simulink model "Flux_Nonsensor"  (R2024a)
settings: Solver=FixedStepDiscrete  StartTime=0.0  StopTime=2  FixedStep=Fixed_Step_Size  RelTol=1e-3
InitFcn:
  | Flux_Nonsensor_data_new
  | 
  | supplyVoltage=30;
values from neighbouring files (symbols this model uses):
  A = 1    [saddleToDuty.m]
  BandwidthCurrentPI = 1256*1.5    (= 1884)    [Flux_Nonsensor_data_new.m]
  Fixed_Step_Size = 1e-6    (= 1e-06)    [Flux_Nonsensor_data_new.m]
  Flux = 0.01837    [Flux_Nonsensor_data_new.m]
  Gamma = mpt.Parameter    [Flux_Nonsensor_data_new.m]
  Ld = 0.0001    [Flux_Nonsensor_data_new.m]
  Lq = 0.0001040    (= 0.000104)    [Flux_Nonsensor_data_new.m]
  Ls = 0.000195185    [Flux_Nonsensor_data_new.m]
  MaxVoltage = 10    [Flux_Nonsensor_data_new.m]
  pll_omega = mpt.Parameter    [Flux_Nonsensor_data_new.m]
  pll_xi = mpt.Parameter    [Flux_Nonsensor_data_new.m]
  PolePairs = 3    [Flux_Nonsensor_data_new.m]
  Rs = 0.02065    [Flux_Nonsensor_data_new.m]
  Speed_Ki = mpt.Parameter    [Flux_Nonsensor_data_new.m]
  Speed_Kp = mpt.Parameter    [Flux_Nonsensor_data_new.m]
  Speed_PI_OutputMax = 8    [Flux_Nonsensor_data_new.m]
  Speed_PI_OutputMin = -8    [Flux_Nonsensor_data_new.m]
  TsBSP = 1e-4    (= 0.0001)    [Flux_Nonsensor_data_new.m]
  TsBSP_MODEL = 2.5e-5    (= 2.5e-05)    [Flux_Nonsensor_data_new.m]
  TsFOC = 1e-4    (= 0.0001)    [Flux_Nonsensor_data_new.m]
undefined symbols (not defined in the file or in its folder): DiscIntNeverNeededParam, magnitude
libraries: slpidlib x3, simulink x2, mcbplantlib x1, spsDCVoltageSourceLib x1, spsSVPWMGenerator2LevelLib x1, spsGroundLib x1, autolibpmsminterior x1, spsPermanentMagnetSynchronousMachineLib x1, spsThreePhaseVIMeasurementLib x1, spsUniversalBridgeLib x1, spspowerguiLib x1
(part 2 of 2)

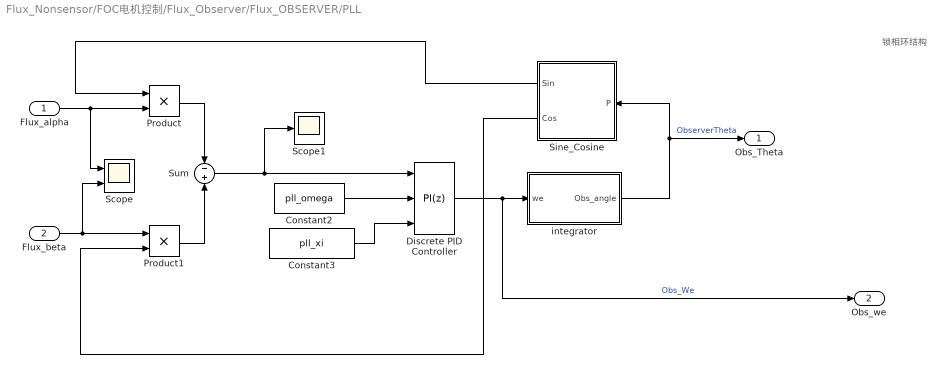
== system Flux_Nonsensor/FOC电机控制/Flux_Observer/Flux_OBSERVER/PLL ==
  note: 锁相环结构
  Flux_alpha : Inport  OutDataTypeStr=single
  Flux_beta : Inport  Port=2  OutDataTypeStr=single
  Constant2 : Constant  Value=pll_omega  OutDataTypeStr=single
  Constant3 : Constant  Value=pll_xi  OutDataTypeStr=single
  Discrete PID Controller : slpidlib/PID Controller  Controller=PI  Form=Parallel  TimeDomain=Discrete-time  UseExternalTs=off  SampleTime=-1  IntegratorMethod=Forward Euler  FilterMethod=Forward Euler  ControllerParametersSource=external  P=2*0.707*1650  I=1650*1650  UseKiTs=off  D=0  UseExternalDerivativeSource=off  N=100  UseFilter=on  TunerSelectOption=Transfer Function Based (PID Tuner App)  ZeroCross=off  InitialConditionSource=internal  InitialConditionForIntegrator=0  InitialConditionForFilter=0  DifferentiatorICPrevScaledInput=0  ExternalReset=none  TrackingMode=off  Kt=1  LimitOutput=on  SatLimitsSource=internal  UpperSaturationLimit=3000*2*pi*PolePairs/60  LowerSaturationLimit=-3000*2*pi*PolePairs/60  LinearizeAsGain=off  AntiWindupMode=clamping  Kb=1  LimitIntegrator=off  UpperIntegratorSaturationLimit=inf  LowerIntegratorSaturationLimit=-inf  POutMin=[]  POutMax=[]  IOutMin=[]  IOutMax=[]  DOutMin=[]  DOutMax=[]  NOutMin=[]  NOutMax=[]  SumOutMin=[]  SumOutMax=[]  SaturationOutMin=[]  SaturationOutMax=[]  PParamMin=[]  PParamMax=[]  IParamMin=[]  IParamMax=[]  DParamMin=[]  DParamMax=[]  NParamMin=[]  NParamMax=[]  KbParamMin=[]  KbParamMax=[]  KtParamMin=[]  KtParamMax=[]  KbOutMin=[]  KbOutMax=[]  KtOutMin=[]  KtOutMax=[]  IntegratorOutMin=[]  IntegratorOutMax=[]  FilterOutMin=[]  FilterOutMax=[]  SumI1OutMin=[]  SumI1OutMax=[]  SumI2OutMin=[]  SumI2OutMax=[]  SumI3OutMin=[]  SumI3OutMax=[]  SumI4OutMin=[]  SumI4OutMax=[]  SumDOutMin=[]  SumDOutMax=[]  DifferentiatorOutMin=[]  DifferentiatorOutMax=[]  FilterDiffOutCoefMin=[]  FilterDiffOutCoefMax=[]  ReciprocalOutMin=[]  ReciprocalOutMax=[]  SumDenOutMin=[]  SumDenOutMax=[]  SumNumOutMin=[]  SumNumOutMax=[]  DivideOutMin=[]  DivideOutMax=[]  UdiffTsProdOutMin=[]  UdiffTsProdOutMax=[]  NTsProdOutMin=[]  NTsProdOutMax=[]  UintegralTsProdOutMin=[]  UintegralTsProdOutMax=[]  UngainTsProdOutMin=[]  UngainTsProdOutMax=[]  ClampingZeroOutDataTypeStr=Inherit: Inherit via back propagation  ClampingZeroOutMin=[]  ClampingZeroOutMax=[]  FilterDenConstantOutDataTypeStr=Inherit: Inherit via back propagation  FilterDenConstantOutMin=[]  FilterDenConstantOutMax=[]  PCopyOutDataTypeStr=Inherit: Inherit via back propagation  PCopyOutMin=[]  PCopyOutMax=[]  NCopyOutDataTypeStr=Inherit: Inherit via back propagation  NCopyOutMin=[]  NCopyOutMax=[]  IntegratorContinuousStateAttributes=''  IntegratorStateMustResolveToSignalObject=off  IntegratorRTWStateStorageClass=Auto  FilterContinuousStateAttributes=''  FilterStateMustResolveToSignalObject=off  FilterRTWStateStorageClass=Auto  ParallelPVariant=ExternalParameters  IdealPVariant=Disabled  IVariant=ExternalParameters  DVariant=Disabled  IntegratorVariant=Discrete  SatVariant=Enabled  AWVariant=DiscClampingParallel  PCopyVariant=Disabled  TRVariant=Disabled  FdbkBlocksVariant=Forward  IdealPFdbkVariant=Disabled  SatFdbkVariant=Disabled  DerivativeFilterVariant=Disabled  NVariant=Disabled  NCopyVariant=Disabled_SignalSpec  FilterICVariant=Disabled  IntegratorICVariant=InternalICs  ExternalResetVariant=Disabled  TRSumVariant=Passthrough  SumFdbkVariant=Disabled  SumVariant=Sum_PI  TsampFilterVariant=InternalTs  TsampNgainVariant=Passthrough  TsampIntegralVariant=Disabled_SignalSpec  ExternalSaturationOutDataTypeStr=Inherit: Same as second input  DerivativeSourceVariant=Disabled
  Product : Product  OutDataTypeStr=single
  Product1 : Product  OutDataTypeStr=single
  Scope : Scope  NumInputPorts=2
  Scope1 : Scope
  Sine_Cosine : Subsystem  TreatAsAtomicUnit=on
      settings: RTWSystemCode=Nonreusable function  RTWFcnNameOpts=Use subsystem name
  Sum : Sum  Inputs=-|+  OutDataTypeStr=single
  integrator : Subsystem
  Obs_Theta : Outport  OutDataTypeStr=single
  Obs_we : Outport  Port=2  OutDataTypeStr=single
  wires:
  Product/1 -> Sum/1
  Product1/1 -> Sum/2
  Sum/1 -> Scope1/1, Discrete PID Controller/1
  Sine_Cosine/2(Cos) -> Product1/2
  Sine_Cosine/1(Sin) -> Product/1
  integrator/1(Obs_angle) -> Obs_Theta/1, Sine_Cosine/1(P)  "ObserverTheta"
  Flux_alpha/1 -> Scope/1, Product/2
  Flux_beta/1 -> Scope/2, Product1/1
  Discrete PID Controller/1 -> Obs_we/1, integrator/1(we)  "Obs_We"
  Constant3/1 -> Discrete PID Controller/3
  Constant2/1 -> Discrete PID Controller/2

== system Flux_Nonsensor/FOC电机控制/Flux_Observer/Flux_OBSERVER/PLL/Sine_Cosine ==
  note: Sine Cosine Coefficients
  P : Inport  OutDataTypeStr=single
  Cos1 : Trigonometry  Operator=cos
  Saturation : Saturate  UpperLimit=2*pi-0.001  LowerLimit=0+0.001  OutDataTypeStr=single
  Scope : Scope  NumInputPorts=2
  Sin1 : Trigonometry
  Sin : Outport  VectorParamsAs1DForOutWhenUnconnected=off
  Cos : Outport  Port=2  VectorParamsAs1DForOutWhenUnconnected=off
  wires:
  P/1 -> Saturation/1  "position"
  Sin1/1 -> Scope/1, Sin/1
  Cos1/1 -> Scope/2, Cos/1
  Saturation/1 -> Cos1/1, Sin1/1

== system Flux_Nonsensor/FOC电机控制/Flux_Observer/Flux_OBSERVER/PLL/integrator ==
  we : Inport  OutDataTypeStr=single
  Angle_Limit : Subsystem
  Sum1 : Sum  Inputs=|++  OutDataTypeStr=single
  Ts : Gain  Gain=TsFOC  OutDataTypeStr=single
  Unit Delay : UnitDelay  SampleTime=-1  HasFrameUpgradeWarning=on
  Obs_angle : Outport  OutDataTypeStr=single
  wires:
  we/1 -> Ts/1
  Ts/1 -> Sum1/1
  Sum1/1 -> Angle_Limit/1(Angle_input)
  Unit Delay/1 -> Obs_angle/1, Sum1/2
  Angle_Limit/1(Angle_output) -> Unit Delay/1

== system Flux_Nonsensor/FOC电机控制/Flux_Observer/Flux_OBSERVER/PLL/integrator/Angle_Limit ==
  Angle_input : Inport
  If Action Subsystem1 : Subsystem  TreatAsAtomicUnit=on
  If Action Subsystem2 : Subsystem  TreatAsAtomicUnit=on
  If Action Subsystem3 : Subsystem  TreatAsAtomicUnit=on
  If1 : If  IfExpression=u1 > 6.283185307  ElseIfExpressions=u1<0
  Merge1 : Merge  Inputs=3
  Angle_output : Outport
  wires:
  If1/2 -> If Action Subsystem3/Action
  If1/1 -> If Action Subsystem2/Action
  If1/3 -> If Action Subsystem1/Action
  Merge1/1 -> Angle_output/1
  If Action Subsystem1/1(Out1) -> Merge1/3
  If Action Subsystem2/1(Out1) -> Merge1/1
  Angle_input/1 -> If Action Subsystem3/1(In1), If Action Subsystem1/1(In1), If Action Subsystem2/1(In1), If1/1
  If Action Subsystem3/1(Out1) -> Merge1/2

== system Flux_Nonsensor/FOC电机控制/Flux_Observer/Flux_OBSERVER/PLL/integrator/Angle_Limit/If Action Subsystem1 ==
  In1 : Inport
  Action Port : ActionPort  ActionPortLabel=else
  Out1 : Outport
  wires:
  In1/1 -> Out1/1

== system Flux_Nonsensor/FOC电机控制/Flux_Observer/Flux_OBSERVER/PLL/integrator/Angle_Limit/If Action Subsystem2 ==
  In1 : Inport
  Action Port : ActionPort  ActionPortLabel=if(u1 > 6.283185307)
  2pi : Constant  Value=2*pi  OutDataTypeStr=single
  Subtract1 : Sum  Inputs=+-  OutDataTypeStr=single
  Out1 : Outport
  wires:
  In1/1 -> Subtract1/1
  Subtract1/1 -> Out1/1
  2pi/1 -> Subtract1/2

== system Flux_Nonsensor/FOC电机控制/Flux_Observer/Flux_OBSERVER/PLL/integrator/Angle_Limit/If Action Subsystem3 ==
  In1 : Inport
  Action Port : ActionPort  ActionPortLabel=elseif(u1<0)
  Angle_offset : Constant  Value=2*pi  OutDataTypeStr=single
  Subtract1 : Sum
  Out1 : Outport
  wires:
  In1/1 -> Subtract1/1
  Subtract1/1 -> Out1/1
  Angle_offset/1 -> Subtract1/2

== matlab function Flux_Nonsensor/FOC电机控制/MATLAB Function ==
  data: saddle1 input; saddle2 input; saddle3 input; frequency input; pwm1 output; deadtime input; pwm1_comp output; pwm2 output; pwm2_comp output; pwm3 output; pwm3_comp output
function [pwm1, pwm1_comp, pwm2, pwm2_comp, pwm3, pwm3_comp] = generatePWMDuty(saddle1, saddle2, saddle3, frequency, deadtime)
    % 参数说明：
    % saddle1, saddle2, saddle3: 输入的三个马鞍波信号（归一化0-1）
    % frequency: PWM 的频率，单位 Hz
    % deadtime: 死区时间，单位 us
    
    % 检查输入信号长度一致性
    if length(saddle1) ~= length(saddle2) || length(saddle2) ~= length(saddle3)
        %error('输入的三个马鞍波信号长度必须一致');
    end
    
    % 设定仿真参数
    Ts = 1e-6; % 仿真步长，1微秒
    T_pwm = 1 / frequency; % PWM周期
    t = (0:length(saddle1)-1) * Ts; % 时间轴与信号点一致
    
    % 生成三角波（0-1归一化）
    triangle = mod(t / T_pwm, 1);
    
    % 比较生成PWM信号
    pwm1 = saddle1 > triangle;
    pwm2 = saddle2 > triangle;
    pwm3 = saddle3 > triangle;
    
    % 生成互补PWM信号
    pwm1_comp = ~pwm1;
    pwm2_comp = ~pwm2;
    pwm3_comp = ~pwm3;
    
    % 添加死区
    deadtime_steps = round(deadtime / (Ts * 1e6)); % 死区转换为步数
    pwm1 = addDeadtime(pwm1, pwm1_comp, deadtime_steps);
    pwm2 = addDeadtime(pwm2, pwm2_comp, deadtime_steps);
    pwm3 = addDeadtime(pwm3, pwm3_comp, deadtime_steps);
    
    % 输出
    pwm1_comp = ~pwm1; % 更新互补波
    pwm2_comp = ~pwm2;
    pwm3_comp = ~pwm3;
end

function pwm_out = addDeadtime(pwm, pwm_comp, deadtime_steps)
    % 为PWM信号添加死区时间
    pwm_out = pwm;
    for i = 1:length(pwm) - deadtime_steps
        if pwm(i) && pwm_comp(i + deadtime_steps)
            pwm_out(i:i + deadtime_steps) = 0;
        end
    end
end

== matlab function Flux_Nonsensor/FOC电机控制/SVPWM MATLAB Function ==
  data: Valpha input single size=1; Tcmp1 output single size=1; Vbeta input single size=1; Tcmp2 output single size=1; Tcmp3 output single size=1; Udc input single size=1; Tpwm input single size=1; sector output single size=1
function [Tcmp1,Tcmp2,Tcmp3,sector] = fcn(Valpha,Vbeta,Udc,Tpwm)
%#codegen

sector = single(0);
Tcmp1 = single(0);
Tcmp2 = single(0);
Tcmp3 = single(0);

%========Parameters statement================

    Vref1 = Vbeta;							                   
    Vref2 = (sqrt(3)*Valpha - Vbeta)/2; 				    
    Vref3 = (-sqrt(3)*Valpha - Vbeta)/2;					
   
 %========Sector calculation=================

  if (Vref1>0)
	   sector = single(1);
  end
  if (Vref2>0)
	   sector = sector+single(2);
  end
  if (Vref3>0)
       sector = sector+single(4);
  end

%======== X Y Z calculation===================

X = sqrt(3)*Vbeta*Tpwm/Udc;
Y = Tpwm/Udc*(3/2*Valpha+sqrt(3)/2*Vbeta);
Z = Tpwm/Udc*(-3/2*Valpha+sqrt(3)/2*Vbeta);	         

%==========Duty ratio calculation================
switch (sector)   
    case 1
        T1 = Z; T2 = Y; 
	case 2
        T1 = Y; T2 = -X; 
	case 3
        T1 = -Z; T2 = X; 
	case 4
        T1 = -X; T2 = Z;
	case 5
        T1 = X; T2 = -Y;
    otherwise
        T1 = -Y; T2 = -Z;
end

if T1+T2 > Tpwm
    T1 = T1/(T1+T2);
    T2 = T2/(T1+T2);
else
    T1 = T1;
    T2 = T2;
end
ta = (Tpwm-(T1+T2))/4.0;
tb = ta+T1/2;
tc = tb+T2/2;

%==========Duty ratio calculation================
switch (sector)
    case 1 
        Tcmp1=tb;
        Tcmp2=ta;
        Tcmp3=tc; 
        
    case 2 
        Tcmp1=ta;
        Tcmp2=tc;
        Tcmp3=tb; 
       
    case 3 
        Tcmp1=ta;
        Tcmp2=tb;
        Tcmp3=tc; 
        
    case 4 
        Tcmp1=tc;
        Tcmp2=tb;
        Tcmp3=ta;
        
    case 5 
        Tcmp1=tc;
        Tcmp2=ta;
        Tcmp3=tb;
        
   case 6
       Tcmp1=tb;
       Tcmp2=tc;
       Tcmp3=ta;
end
end

== matlab function Flux_Nonsensor/FOC电机控制/MATLAB Function1 ==
  data: Valpha input; duty_3 output; Vbeta input; Vdc input
function duty_3 = svGen(Valpha,Vbeta,Vdc)
Valpha_Pu = Valpha/Vdc;
Vbeta_Pu = Vbeta/Vdc;
Vabc_Pu = zeros(3,1);
duty = zeros(3,1);

Vabc_Pu(1) = Valpha_Pu;
Vabc_Pu(2) = -0.5*Valpha_Pu + sqrt(3)/2 * Vbeta_Pu;
Vabc_Pu(3) = -0.5*Valpha_Pu - sqrt(3)/2 * Vbeta_Pu;

Vmax_Pu = max(Vabc_Pu);
Vmin_Pu = min(Vabc_Pu);

Vcom_Pu =0.5 *(Vmax_Pu + Vmin_Pu);

duty(1) = Vabc_Pu(1) - Vcom_Pu + 0.5;
duty(2) = Vabc_Pu(2) - Vcom_Pu + 0.5;
duty(3) = Vabc_Pu(3) - Vcom_Pu + 0.5;
duty_3 = duty;

== matlab function Flux_Nonsensor/MATLAB Function ==
  data: waveA input; pwmHighA output; waveB input; waveC input; samplingInterval input; switchFreq input; deadTime input; pwmLowA output; pwmHighB output; pwmLowB output; pwmHighC output; pwmLowC output
function [pwmHighA, pwmLowA, pwmHighB, pwmLowB, pwmHighC, pwmLowC] = generatePWM6(waveA, waveB, waveC, samplingInterval, switchFreq, deadTime)
    % 参数说明：
    % waveA, waveB, waveC: 输入的三个马鞍波信号 (离散数组)
    % samplingInterval: 最小采样间隔（秒），如 100e-6
    % switchFreq: MOSFET 切换频率 (Hz)
    % deadTime: 死区时间（秒），如 1e-6

    % 计算 PWM 的基准周期
    pwmPeriod = 1 / switchFreq;        % PWM周期 (秒)
    samplesPerCycle = round(pwmPeriod / samplingInterval); % 每个周期的采样点数
    deadSamples = round(deadTime / samplingInterval);      % 死区对应的采样点数

    % 将输入波形归一化到 [0, 1] 区间
    waveA = normalizeWave(waveA);
    waveB = normalizeWave(waveB);
    waveC = normalizeWave(waveC);

    % 生成每对PWM波形
    [pwmHighA, pwmLowA] = createPWM(waveA, samplesPerCycle, deadSamples);
    [pwmHighB, pwmLowB] = createPWM(waveB, samplesPerCycle, deadSamples);
    [pwmHighC, pwmLowC] = createPWM(waveC, samplesPerCycle, deadSamples);
end

function normalizedWave = normalizeWave(wave)
    % 将波形归一化到 [0, 1] 区间
    minVal = min(wave);
    maxVal = max(wave);
    normalizedWave = (wave - minVal) / (maxVal - minVal);
end

function [pwmHigh, pwmLow] = createPWM(wave, samplesPerCycle, deadSamples)
    % 根据输入波形生成一对互补PWM信号
    pwmHigh = zeros(size(wave));
    pwmLow = zeros(size(wave));
    threshold = 0.5;  % 比较的参考值（归一化中点）

    % 遍历波形生成PWM
    for i = 1:length(wave)
        % PWM 高电平
        if mod(i, samplesPerCycle) <= wave(i) * samplesPerCycle
            pwmHigh(i) = 1;
        else
            pwmHigh(i) = 0;
        end

        % 加入死区处理
        if i > deadSamples && pwmHigh(i - deadSamples) == 1
            pwmHigh(i) = 0;
        end

        % PWM 低电平为互补
        pwmLow(i) = ~pwmHigh(i);

        % 死区时间影响低电平
        if i > deadSamples && pwmLow(i - deadSamples) == 1
            pwmLow(i) = 0;
        end
    end
end

== matlab function Flux_Nonsensor/MATLAB Function1 ==
  data: input_waveforms input; pwm_signals output; sampling_interval input; switching_frequency input; dead_time_us input
function pwm_signals = generate_pwm(input_waveforms, sampling_interval, switching_frequency, dead_time_us)
%#codegen

    % 参数验证
    if size(input_waveforms, 2) ~= 3
        error('Input must contain three waveforms with phase shift of 120 degrees each.');
    end
    
    % 常量计算
    pwm_period = 1 / switching_frequency; % PWM周期 (秒)
    dead_time = dead_time_us * 1e-6;      % 死区时间 (秒)
    num_samples = size(input_waveforms, 1); % 输入信号样本数
    
    % 初始化输出信号
    pwm_signals = zeros(num_samples, 6); % 每相互补，6路信号
    
    % 归一化输入波形到[0, 1]
    normalized_waveforms = (input_waveforms - min(input_waveforms, [], 1)) ./ ...
                           (max(input_waveforms, [], 1) - min(input_waveforms, [], 1));
    
    % 逐样本生成PWM信号
    for i = 1:num_samples
        for phase = 1:3
            % 计算占空比
            duty_cycle = normalized_waveforms(i, phase);
            
            % 计算高低信号时间
            high_time = duty_cycle * pwm_period;
            low_time = pwm_period - high_time;
            
            % 添加死区
            if high_time > dead_time && low_time > dead_time
                pwm_signals(i, 2*phase-1) = 1; % 高边PWM信号
                pwm_signals(i, 2*phase) = 0;   % 低边PWM信号
            else
                pwm_signals(i, 2*phase-1) = 0; % 死区内信号关断
                pwm_signals(i, 2*phase) = 0;
            end
        end
    end
end

== matlab function Flux_Nonsensor/FOC电机控制/MATLAB Function2 ==
  data: input_signal input; pwm_signals output
function pwm_signals = generate_pwm(input_signal)
% Generate 6 complementary PWM signals based on a saddle wave input.
% Input:
%   input_signal - Normalized discrete saddle wave signal, phase-shifted by 120 degrees.
% Output:
%   pwm_signals - Matrix of 6 PWM signals for the MCU (3 complementary pairs).

% Parameters
pwm_period = 2400;  % PWM max count value (center-aligned)
pwm_mid = pwm_period / 2;  % Center count value

% Scale input signal to PWM range
scaled_signal = pwm_mid * (1 + input_signal); % Scale to 0 to 2400

% Ensure the scaled signal stays within the bounds
scaled_signal(scaled_signal > pwm_period) = pwm_period;
scaled_signal(scaled_signal < 0) = 0;

% Generate the six PWM signals
% Three phases (A, B, C) are phase-shifted by 120 degrees each
phase_A = scaled_signal;
phase_B = circshift(scaled_signal, [0, round(length(scaled_signal) / 3)]); % 120-degree shift
phase_C = circshift(scaled_signal, [0, 2 * round(length(scaled_signal) / 3)]); % 240-degree shift

% Complementary signals
complementary_A = pwm_period - phase_A;
complementary_B = pwm_period - phase_B;
complementary_C = pwm_period - phase_C;

% Combine signals into a matrix for output
pwm_signals = [phase_A; complementary_A; phase_B; complementary_B; phase_C; complementary_C];
end
